simulink model "Test_mcb_pmsm_foc_sim_RL"  (R2020b)
settings: Solver=FixedStepDiscrete  StartTime=0.0  StopTime=6  RelTol=1e-3  EnableMultiTasking=on
values from neighbouring files (symbols this model uses):
  coeff_d = readmatrix('C:\Users\terzo\LearningX\advanced_ML\model_tree\output_d\coeff.txt')    [readtrees.m]
  coeff_q = readmatrix('C:\Users\terzo\LearningX\advanced_ML\model_tree\output_q\coeff.txt')    [readtrees.m]
  index_d = readmatrix('C:\Users\terzo\LearningX\advanced_ML\model_tree\output_d\index.txt')    [readtrees.m]
  index_q = readmatrix('C:\Users\terzo\LearningX\advanced_ML\model_tree\output_q\index.txt')    [readtrees.m]
  intercept_d = readmatrix('C:\Users\terzo\LearningX\advanced_ML\model_tree\output_d\intercept.txt')    [readtrees.m]
  intercept_q = readmatrix('C:\Users\terzo\LearningX\advanced_ML\model_tree\output_q\intercept.txt')    [readtrees.m]
  inverter = mcb_SetInverterParameters_RL('BoostXL-DRV8305')    [sim_data.m]
  maxAngleIn = 1    [sim_data.m]
  MechOfstInputType = pmsm.p    [sim_data.m]
  PI_params = mcb.internal.SetControllerParameters(pmsm,inverter,PU_System,T_pwm,Ts,Ts_speed)    [sim_data.m]
  PU_System = mcb_SetPUSystem_RL(pmsm,inverter)    [sim_data.m]
  threshold_d = readmatrix('C:\Users\terzo\LearningX\advanced_ML\model_tree\output_d\treshold.txt')    [readtrees.m]
  threshold_q = readmatrix('C:\Users\terzo\LearningX\advanced_ML\model_tree\output_q\treshold.txt')    [readtrees.m]
  Ts_motor = T_pwm/2    (= 0.0001)    [sim_data.m]
  Ts_simulink = T_pwm/2    (= 0.0001)    [sim_data.m]
  Ts_speed = 10*Ts    (= 0.002)    [sim_data.m]
undefined symbols (not defined in the file or in its folder): DiscIntNeverNeededParam, pmsm
libraries: mcbcontrolslib x22, mcbpositiondecoderlib x6, simulink x4, mcbplantlib x2, autolibpmsmexterior x2, rllib x1
(part 2 of 2)

== matlab function Test_mcb_pmsm_foc_sim_RL/Current Control/Control_System/Closed Loop Control/Reinforcement Learning/tree_d ==
  data: u input; y output size=1; coeff_d parameter; intercept_d parameter; index_d parameter; threshold_d parameter
function y = fcn(u, coeff_d, intercept_d, index_d, threshold_d)
% i = 1;
% predicted = dnodeMean(i);
% while dcutePredictorIndex(i) ~= 0
%     if u(dcutePredictorIndex(i)) < dcut_point(i)
%         i = dchildren(i, 1);
%     else
%         i = dchildren(i, 2);
%     end
%     
%     predicted = dnodeMean(i);
% end   
mt_d = ModelTree(coeff_d, intercept_d, index_d, threshold_d);
y = mt_d.predict(u');

== matlab function Test_mcb_pmsm_foc_sim_RL/Current Control/Control_System/Closed Loop Control/Reinforcement Learning/tree_q ==
  data: u input; y output size=1; coeff_q parameter; intercept_q parameter; index_q parameter; threshold_q parameter
function y = fcn(u, coeff_q, intercept_q, index_q, threshold_q)
% i = 1;
% predicted = qnodeMean(i);
% while qcutePredictorIndex(i) ~= 0
%     if u(qcutePredictorIndex(i)) < qcut_point(i)
%         i = qchildren(i, 1);
%     else
%         i = qchildren(i, 2);
%     end
%     
%     predicted = qnodeMean(i);
% end
mt_q = ModelTree(coeff_q, intercept_q, index_q, threshold_q);
y = mt_q.predict(u');
